simulink model "TPS_Characteristic"  (R2024b)
settings: Solver=VariableStepAuto  StartTime=0.0  StopTime=10.0  RelTol=1e-3
settings Model: Creator=MOHAMED  LastModifiedBy=MOHAMED

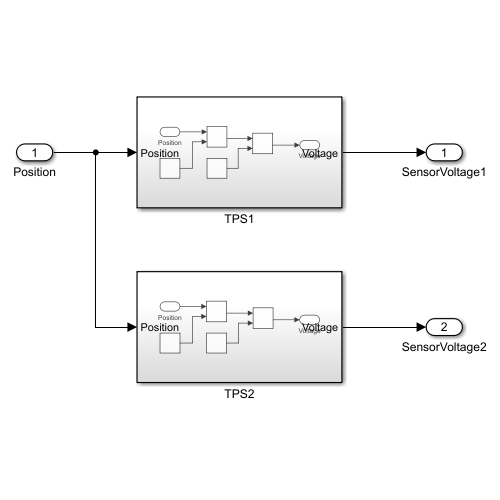
[thumbnail: Simulink's stored preview of the top-level diagram]
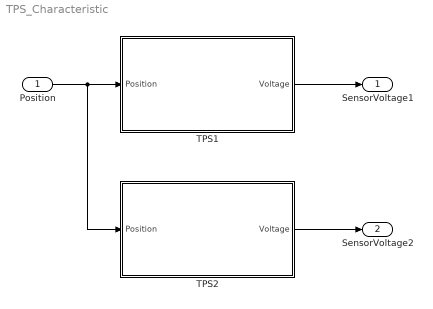
== system TPS_Characteristic ==
  Position : Inport
  TPS1 : Subsystem
  TPS2 : Subsystem
  SensorVoltage1 : Outport
  SensorVoltage2 : Outport  Port=2
  wires:
  Position/1 -> TPS2/1(Position), TPS1/1(Position)
  TPS2/1(Voltage) -> SensorVoltage2/1
  TPS1/1(Voltage) -> SensorVoltage1/1

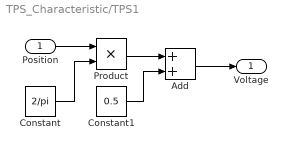
== system TPS_Characteristic/TPS1 ==
  Position : Inport
  Add : Sum
  Constant : Constant  Value=2/pi
  Constant1 : Constant  Value=0.5
  Product : Product
  Voltage : Outport
  wires:
  Position/1 -> Product/1
  Product/1 -> Add/1
  Constant/1 -> Product/2
  Add/1 -> Voltage/1
  Constant1/1 -> Add/2

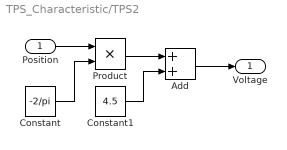
== system TPS_Characteristic/TPS2 ==
  Position : Inport
  Add : Sum
  Constant : Constant  Value=-2/pi
  Constant1 : Constant  Value=4.5
  Product : Product
  Voltage : Outport
  wires:
  Constant1/1 -> Add/2
  Add/1 -> Voltage/1
  Constant/1 -> Product/2
  Product/1 -> Add/1
  Position/1 -> Product/1
